simulink model "plant_n"  (R2023a)
settings: Solver=FixedStepAuto  StartTime=0.0  StopTime=200  FixedStep=0.01  RelTol=1e-3
values from neighbouring files (symbols this model uses):
  filter_3 = conv([0.1,1],conv([0.1 1],[0.1 1]))    [main_proj.m]
  filter_x = conv([0.7,1],conv([0.7 1],[0.7 1]))    [main_proj.m]
  kd = 1.117    [main_proj.m]
  ki = 4.47    [main_proj.m]
  kp = 5.366    [main_proj.m]
libraries: neural x772, slpidlib x6
(part 15 of 26)

== system plant_n/NARX Neural Network m8 gud (solution 2)/Layer 1/Delays 2 ==
  "p{1}" : Inport  PortDimensions=1  SampleTime=0.01
      mask Display: e = 0.06;c1 = [120 230 180]/255;c2 = ([120 230 180]+0)/(256+128);c3 = ([120 230 180]+128)/(256+128);patch([0 1 1 0],[0 0 1 1],c1);patch([0 1 1 1-e 1-e 0+e],[0 0 1 1-e 0+e 0+e],c2);patch([0 0 1 1-e 0+e 0+e],[0 1 1 1-e 1-e 0+e],c3);plot([0 1 1 0 0],[0 0 1 1 0]);
  Delay 1 : UnitDelay  InitialCondition=ai_layer_2_delayed_1  SampleTime=0.01
      mask Display: e = 0.06;c1 = [120 150 230]/255;c2 = ([120 150 230]+0)/383;c3 = ([120 150 230]+128)/383;patch([0 1 1 0],[0 0 1 1],c1);patch([0 1 1 1-e 1-e 0+e],[0 0 1 1-e 0+e 0+e],c2);patch([0 0 1 1-e 0+e 0+e],[0 1 1 1-e 1-e 0+e],c3);plot([0 1 1 0 0],[0 0 1 1 0]);disp('D')
  Delay 10 : UnitDelay  InitialCondition=ai_layer_2_delayed_10  SampleTime=0.01
      mask Display: e = 0.06;c1 = [120 150 230]/255;c2 = ([120 150 230]+0)/383;c3 = ([120 150 230]+128)/383;patch([0 1 1 0],[0 0 1 1],c1);patch([0 1 1 1-e 1-e 0+e],[0 0 1 1-e 0+e 0+e],c2);patch([0 0 1 1-e 0+e 0+e],[0 1 1 1-e 1-e 0+e],c3);plot([0 1 1 0 0],[0 0 1 1 0]);disp('D')
  Delay 11 : UnitDelay  InitialCondition=ai_layer_2_delayed_11  SampleTime=0.01
      mask Display: e = 0.06;c1 = [120 150 230]/255;c2 = ([120 150 230]+0)/383;c3 = ([120 150 230]+128)/383;patch([0 1 1 0],[0 0 1 1],c1);patch([0 1 1 1-e 1-e 0+e],[0 0 1 1-e 0+e 0+e],c2);patch([0 0 1 1-e 0+e 0+e],[0 1 1 1-e 1-e 0+e],c3);plot([0 1 1 0 0],[0 0 1 1 0]);disp('D')
  Delay 12 : UnitDelay  InitialCondition=ai_layer_2_delayed_12  SampleTime=0.01
      mask Display: e = 0.06;c1 = [120 150 230]/255;c2 = ([120 150 230]+0)/383;c3 = ([120 150 230]+128)/383;patch([0 1 1 0],[0 0 1 1],c1);patch([0 1 1 1-e 1-e 0+e],[0 0 1 1-e 0+e 0+e],c2);patch([0 0 1 1-e 0+e 0+e],[0 1 1 1-e 1-e 0+e],c3);plot([0 1 1 0 0],[0 0 1 1 0]);disp('D')
  Delay 2 : UnitDelay  InitialCondition=ai_layer_2_delayed_2  SampleTime=0.01
      mask Display: e = 0.06;c1 = [120 150 230]/255;c2 = ([120 150 230]+0)/383;c3 = ([120 150 230]+128)/383;patch([0 1 1 0],[0 0 1 1],c1);patch([0 1 1 1-e 1-e 0+e],[0 0 1 1-e 0+e 0+e],c2);patch([0 0 1 1-e 0+e 0+e],[0 1 1 1-e 1-e 0+e],c3);plot([0 1 1 0 0],[0 0 1 1 0]);disp('D')
  Delay 3 : UnitDelay  InitialCondition=ai_layer_2_delayed_3  SampleTime=0.01
      mask Display: e = 0.06;c1 = [120 150 230]/255;c2 = ([120 150 230]+0)/383;c3 = ([120 150 230]+128)/383;patch([0 1 1 0],[0 0 1 1],c1);patch([0 1 1 1-e 1-e 0+e],[0 0 1 1-e 0+e 0+e],c2);patch([0 0 1 1-e 0+e 0+e],[0 1 1 1-e 1-e 0+e],c3);plot([0 1 1 0 0],[0 0 1 1 0]);disp('D')
  Delay 4 : UnitDelay  InitialCondition=ai_layer_2_delayed_4  SampleTime=0.01
      mask Display: e = 0.06;c1 = [120 150 230]/255;c2 = ([120 150 230]+0)/383;c3 = ([120 150 230]+128)/383;patch([0 1 1 0],[0 0 1 1],c1);patch([0 1 1 1-e 1-e 0+e],[0 0 1 1-e 0+e 0+e],c2);patch([0 0 1 1-e 0+e 0+e],[0 1 1 1-e 1-e 0+e],c3);plot([0 1 1 0 0],[0 0 1 1 0]);disp('D')
  Delay 5 : UnitDelay  InitialCondition=ai_layer_2_delayed_5  SampleTime=0.01
      mask Display: e = 0.06;c1 = [120 150 230]/255;c2 = ([120 150 230]+0)/383;c3 = ([120 150 230]+128)/383;patch([0 1 1 0],[0 0 1 1],c1);patch([0 1 1 1-e 1-e 0+e],[0 0 1 1-e 0+e 0+e],c2);patch([0 0 1 1-e 0+e 0+e],[0 1 1 1-e 1-e 0+e],c3);plot([0 1 1 0 0],[0 0 1 1 0]);disp('D')
  Delay 6 : UnitDelay  InitialCondition=ai_layer_2_delayed_6  SampleTime=0.01
      mask Display: e = 0.06;c1 = [120 150 230]/255;c2 = ([120 150 230]+0)/383;c3 = ([120 150 230]+128)/383;patch([0 1 1 0],[0 0 1 1],c1);patch([0 1 1 1-e 1-e 0+e],[0 0 1 1-e 0+e 0+e],c2);patch([0 0 1 1-e 0+e 0+e],[0 1 1 1-e 1-e 0+e],c3);plot([0 1 1 0 0],[0 0 1 1 0]);disp('D')
  Delay 7 : UnitDelay  InitialCondition=ai_layer_2_delayed_7  SampleTime=0.01
      mask Display: e = 0.06;c1 = [120 150 230]/255;c2 = ([120 150 230]+0)/383;c3 = ([120 150 230]+128)/383;patch([0 1 1 0],[0 0 1 1],c1);patch([0 1 1 1-e 1-e 0+e],[0 0 1 1-e 0+e 0+e],c2);patch([0 0 1 1-e 0+e 0+e],[0 1 1 1-e 1-e 0+e],c3);plot([0 1 1 0 0],[0 0 1 1 0]);disp('D')
  Delay 8 : UnitDelay  InitialCondition=ai_layer_2_delayed_8  SampleTime=0.01
      mask Display: e = 0.06;c1 = [120 150 230]/255;c2 = ([120 150 230]+0)/383;c3 = ([120 150 230]+128)/383;patch([0 1 1 0],[0 0 1 1],c1);patch([0 1 1 1-e 1-e 0+e],[0 0 1 1-e 0+e 0+e],c2);patch([0 0 1 1-e 0+e 0+e],[0 1 1 1-e 1-e 0+e],c3);plot([0 1 1 0 0],[0 0 1 1 0]);disp('D')
  Delay 9 : UnitDelay  InitialCondition=ai_layer_2_delayed_9  SampleTime=0.01
      mask Display: e = 0.06;c1 = [120 150 230]/255;c2 = ([120 150 230]+0)/383;c3 = ([120 150 230]+128)/383;patch([0 1 1 0],[0 0 1 1],c1);patch([0 1 1 1-e 1-e 0+e],[0 0 1 1-e 0+e 0+e],c2);patch([0 0 1 1-e 0+e 0+e],[0 1 1 1-e 1-e 0+e],c3);plot([0 1 1 0 0],[0 0 1 1 0]);disp('D')
  mux : Mux  Inputs=12
      mask Display: e = 0.06;c1 = [120 150 230]/255;c2 = ([120 150 230]+0)/383;c3 = ([120 150 230]+128)/383;patch([0 1 1 0],[0 0 1 1],c1);patch([0 1 1 1-e 1-e 0+e],[0 0 1 1-e 0+e 0+e],c2);patch([0 0 1 1-e 0+e 0+e],[0 1 1 1-e 1-e 0+e],c3);plot([0 1 1 0 0],[0 0 1 1 0]);disp('Mux')
  "pd{1,2}" : Outport
      mask Display: e = 0.06;c1 = [120 230 180]/255;c2 = ([120 230 180]+0)/(256+128);c3 = ([120 230 180]+128)/(256+128);patch([0 1 1 0],[0 0 1 1],c1);patch([0 1 1 1-e 1-e 0+e],[0 0 1 1-e 0+e 0+e],c2);patch([0 0 1 1-e 0+e 0+e],[0 1 1 1-e 1-e 0+e],c3);plot([0 1 1 0 0],[0 0 1 1 0]);
  wires:
  "p{1}"/1 -> Delay 1/1
  Delay 1/1 -> Delay 2/1, mux/1
  Delay 2/1 -> Delay 3/1, mux/2
  Delay 3/1 -> Delay 4/1, mux/3
  Delay 4/1 -> Delay 5/1, mux/4
  Delay 5/1 -> Delay 6/1, mux/5
  Delay 6/1 -> Delay 7/1, mux/6
  Delay 7/1 -> Delay 8/1, mux/7
  Delay 8/1 -> Delay 9/1, mux/8
  Delay 9/1 -> Delay 10/1, mux/9
  Delay 10/1 -> Delay 11/1, mux/10
  Delay 11/1 -> Delay 12/1, mux/11
  Delay 12/1 -> mux/12
  mux/1 -> "pd{1,2}"/1

== system plant_n/NARX Neural Network m8 gud (solution 2)/Layer 1/IW{1,1} ==
  "pd{1,1}" : Inport  PortDimensions=12  SampleTime=0.01
      mask Display: e = 0.06;c1 = [120 230 180]/255;c2 = ([120 230 180]+0)/(256+128);c3 = ([120 230 180]+128)/(256+128);patch([0 1 1 0],[0 0 1 1],c1);patch([0 1 1 1-e 1-e 0+e],[0 0 1 1-e 0+e 0+e],c2);patch([0 0 1 1-e 0+e 0+e],[0 1 1 1-e 1-e 0+e],c3);plot([0 1 1 0 0],[0 0 1 1 0]);
  "IW{1,1}(1,:)'" : Constant  Value=[-0.56334830130879154364009764321963302791118621826171875;-0.357985255096524290774340215648408047854900360107421875;0.283427998989764062809371125695179216563701629638671875;-0.52727885493944259831522458625840954482555389404296875;-0.278331944433723055265517132284003309905529022216796875;-0.6037598769818128818798186330241151154041290283203125;-0.252123927832144156813143354156636632978916168212890625;0.28838201323591317049022109131328761577606201171875;-0.463874462662791253730887319761677645146846771240234375;0.27896573584558381764253454093704931437969207763671875;0.50570674204775212245976945268921554088592529296875;-0.007390079131495852320099526622243502060882747173309326171875]
      mask Display: e = 0.06;c1 = [120 150 230]/255;c2 = ([120 150 230]+0)/383;c3 = ([120 150 230]+128)/383;patch([0 1 1 0],[0 0 1 1],c1);patch([0 1 1 1-e 1-e 0+e],[0 0 1 1-e 0+e 0+e],c2);patch([0 0 1 1-e 0+e 0+e],[0 1 1 1-e 1-e 0+e],c3);plot([0 1 1 0 0],[0 0 1 1 0]);disp('Weights');
  "IW{1,1}(10,:)'" : Constant  Value=[-0.690275840744874802368258315254934132099151611328125;-0.79728617428333803385243072625598870217800140380859375;0.177674477339559488964226829921244643628597259521484375;0.09590570580940356582022587872415897436439990997314453125;-0.28801320297100974077153523467131890356540679931640625;-0.6833243170596807747330103666172362864017486572265625;-0.22435716680905526398959182188264094293117523193359375;-0.6840716937023392230088347787386737763881683349609375;-0.475131576981321190888962746612378396093845367431640625;-0.12182823067504509884084740178877837024629116058349609375;0.093487293354278244716937251723720692098140716552734375;0.74502502276723092666799175276537425816059112548828125]
      mask Display: e = 0.06;c1 = [120 150 230]/255;c2 = ([120 150 230]+0)/383;c3 = ([120 150 230]+128)/383;patch([0 1 1 0],[0 0 1 1],c1);patch([0 1 1 1-e 1-e 0+e],[0 0 1 1-e 0+e 0+e],c2);patch([0 0 1 1-e 0+e 0+e],[0 1 1 1-e 1-e 0+e],c3);plot([0 1 1 0 0],[0 0 1 1 0]);disp('Weights');
  "IW{1,1}(11,:)'" : Constant  Value=[0.020807334832183312089970428360174992121756076812744140625;-0.72362889068850300144930542955989949405193328857421875;-0.955254334663456550202909056679345667362213134765625;-0.204760678764603853974080038824467919766902923583984375;0.371667191189833878706139103087480179965496063232421875;-0.42938605762169246293780133783002384006977081298828125;-0.09146518961475048892229011698873364366590976715087890625;0.7516682707084567649502560016117058694362640380859375;0.722135567066211958575649987324140965938568115234375;0.2184070815776478491354595234952284954488277435302734375;0.69775866315792012262164689673227258026599884033203125;-0.8721778633994456964018127109738998115062713623046875]
      mask Display: e = 0.06;c1 = [120 150 230]/255;c2 = ([120 150 230]+0)/383;c3 = ([120 150 230]+128)/383;patch([0 1 1 0],[0 0 1 1],c1);patch([0 1 1 1-e 1-e 0+e],[0 0 1 1-e 0+e 0+e],c2);patch([0 0 1 1-e 0+e 0+e],[0 1 1 1-e 1-e 0+e],c3);plot([0 1 1 0 0],[0 0 1 1 0]);disp('Weights');
  "IW{1,1}(12,:)'" : Constant  Value=[-1.057018932574201652840883980388753116130828857421875;0.1693893839232068210254311679818783886730670928955078125;-0.85044934461662291536043767337105236947536468505859375;0.75838542598846381270760730330948717892169952392578125;0.50790235655985827012415256831445731222629547119140625;-0.0171384088579385092387941114111526985652744770050048828125;-0.428656473069752019799949493972235359251499176025390625;-0.16818090949152197932647823108709417283535003662109375;-0.8651226870069035346233476957422681152820587158203125;-0.5193860764043047861804325293633155524730682373046875;1.0594564649420614710351173926028423011302947998046875;-0.1817459257744392930877808112200000323355197906494140625]
      mask Display: e = 0.06;c1 = [120 150 230]/255;c2 = ([120 150 230]+0)/383;c3 = ([120 150 230]+128)/383;patch([0 1 1 0],[0 0 1 1],c1);patch([0 1 1 1-e 1-e 0+e],[0 0 1 1-e 0+e 0+e],c2);patch([0 0 1 1-e 0+e 0+e],[0 1 1 1-e 1-e 0+e],c3);plot([0 1 1 0 0],[0 0 1 1 0]);disp('Weights');
  "IW{1,1}(13,:)'" : Constant  Value=[-0.585951041167996233838266562088392674922943115234375;0.716915749185477846339153984445147216320037841796875;-0.23957537814192109149047382743447087705135345458984375;-0.8104595833058401144199933696654625236988067626953125;-0.30478478512946394207716593882651068270206451416015625;0.81104511509295296178834178135730326175689697265625;0.64501496872723074194055925545399077236652374267578125;-0.07076557953330718520046360708874999545514583587646484375;0.107786241446574726499108010102645494043827056884765625;0.262021628214974822146388078181189484894275665283203125;0.2077129224946279439922847132038441486656665802001953125;-0.33823196160467261517368342538247816264629364013671875]
      mask Display: e = 0.06;c1 = [120 150 230]/255;c2 = ([120 150 230]+0)/383;c3 = ([120 150 230]+128)/383;patch([0 1 1 0],[0 0 1 1],c1);patch([0 1 1 1-e 1-e 0+e],[0 0 1 1-e 0+e 0+e],c2);patch([0 0 1 1-e 0+e 0+e],[0 1 1 1-e 1-e 0+e],c3);plot([0 1 1 0 0],[0 0 1 1 0]);disp('Weights');
  "IW{1,1}(14,:)'" : Constant  Value=[-0.021926861772730621424898345139808952808380126953125;0.8906753535205587102296931334421969950199127197265625;-0.36976128212221792690428401328972540795803070068359375;-0.345367710616706846682433251771726645529270172119140625;-0.768790324260997248728699560160748660564422607421875;-0.219877322789279794346128937831963412463665008544921875;0.6049218279495220951247347329626791179180145263671875;-0.4412884606493763239853933555423282086849212646484375;0.05255967818845840022756732423658831976354122161865234375;-0.45907623086972570991548536767368204891681671142578125;0.6549992864126437108751588311861269176006317138671875;0.488129180308522148123984152334742248058319091796875]
      mask Display: e = 0.06;c1 = [120 150 230]/255;c2 = ([120 150 230]+0)/383;c3 = ([120 150 230]+128)/383;patch([0 1 1 0],[0 0 1 1],c1);patch([0 1 1 1-e 1-e 0+e],[0 0 1 1-e 0+e 0+e],c2);patch([0 0 1 1-e 0+e 0+e],[0 1 1 1-e 1-e 0+e],c3);plot([0 1 1 0 0],[0 0 1 1 0]);disp('Weights');
  "IW{1,1}(15,:)'" : Constant  Value=[0.46117641601221526226339619825012050569057464599609375;-0.0895345461376331475111811641909298487007617950439453125;0.328264117492681528620579456401173956692218780517578125;0.511917503541946761203007554286159574985504150390625;-0.801266579608470141948828313616104423999786376953125;0.451910735167512012111501462641172111034393310546875;-0.2188741480298032893170301349528017453849315643310546875;-0.6286657891340030612781220042961649596691131591796875;0.8327123535010105825904247467406094074249267578125;0.18255510716111655877824659910402260720729827880859375;-0.7387495430428596687733033832046203315258026123046875;-0.3072498793567366437429200232145376503467559814453125]
      mask Display: e = 0.06;c1 = [120 150 230]/255;c2 = ([120 150 230]+0)/383;c3 = ([120 150 230]+128)/383;patch([0 1 1 0],[0 0 1 1],c1);patch([0 1 1 1-e 1-e 0+e],[0 0 1 1-e 0+e 0+e],c2);patch([0 0 1 1-e 0+e 0+e],[0 1 1 1-e 1-e 0+e],c3);plot([0 1 1 0 0],[0 0 1 1 0]);disp('Weights');
  "IW{1,1}(2,:)'" : Constant  Value=[0.0787588482440988169042128674846026115119457244873046875;-0.71485237410952573444689051029854454100131988525390625;-0.261021462395077563645173768236418254673480987548828125;-0.77190171434430976393770151844364590942859649658203125;0.6192120004761527685133160048280842602252960205078125;0.276209900461571955521122845311765559017658233642578125;0.1564198465414966821018794007613905705511569976806640625;0.86245245324036023948366391778108663856983184814453125;-0.029228672295336245723351709102644235827028751373291015625;-0.29333393668341434246116250506020151078701019287109375;0.6675369234504946458486074334359727799892425537109375;-0.6078291827270627667445523911737836897373199462890625]
      mask Display: e = 0.06;c1 = [120 150 230]/255;c2 = ([120 150 230]+0)/383;c3 = ([120 150 230]+128)/383;patch([0 1 1 0],[0 0 1 1],c1);patch([0 1 1 1-e 1-e 0+e],[0 0 1 1-e 0+e 0+e],c2);patch([0 0 1 1-e 0+e 0+e],[0 1 1 1-e 1-e 0+e],c3);plot([0 1 1 0 0],[0 0 1 1 0]);disp('Weights');
  "IW{1,1}(3,:)'" : Constant  Value=[-0.76808344267437067554027407823014073073863983154296875;-0.55038788676150252054952716207480989396572113037109375;0.77459185718728151837098039322881959378719329833984375;-0.499350522556929854456342354751541279256343841552734375;-0.908047325048035869343721060431562364101409912109375;-0.287074786361956768576675358417560346424579620361328125;0.6404765001640833066431923725758679211139678955078125;0.78235408277472651139561321542714722454547882080078125;0.5997842926650067685301337405689992010593414306640625;-0.486908024680651141391507508160430006682872772216796875;0.62504559351542832157377915791585110127925872802734375;-0.1936118783901183137974300052519538439810276031494140625]
      mask Display: e = 0.06;c1 = [120 150 230]/255;c2 = ([120 150 230]+0)/383;c3 = ([120 150 230]+128)/383;patch([0 1 1 0],[0 0 1 1],c1);patch([0 1 1 1-e 1-e 0+e],[0 0 1 1-e 0+e 0+e],c2);patch([0 0 1 1-e 0+e 0+e],[0 1 1 1-e 1-e 0+e],c3);plot([0 1 1 0 0],[0 0 1 1 0]);disp('Weights');
  "IW{1,1}(4,:)'" : Constant  Value=[-0.82639420868754076554552057132241316139698028564453125;-0.276346036675341577559805728014907799661159515380859375;-0.54739563886299269501733988363412208855152130126953125;0.032969016201114260955495893767874804325401782989501953125;0.342569758428644621783831780703621916472911834716796875;-0.33994997710060104179063955598394386470317840576171875;0.91375881388352431233812467326060868799686431884765625;-0.331584671920007900691729219033732078969478607177734375;0.36714835048246918791647885882412083446979522705078125;-0.0846176892761831833666974489460699260234832763671875;-0.92592303920993701549235765924095176160335540771484375;-0.93601802735372918728984359404421411454677581787109375]
      mask Display: e = 0.06;c1 = [120 150 230]/255;c2 = ([120 150 230]+0)/383;c3 = ([120 150 230]+128)/383;patch([0 1 1 0],[0 0 1 1],c1);patch([0 1 1 1-e 1-e 0+e],[0 0 1 1-e 0+e 0+e],c2);patch([0 0 1 1-e 0+e 0+e],[0 1 1 1-e 1-e 0+e],c3);plot([0 1 1 0 0],[0 0 1 1 0]);disp('Weights');
  "IW{1,1}(5,:)'" : Constant  Value=[0.91859542281127726237599517844500951468944549560546875;-0.07037748658693605829927975037207943387329578399658203125;-0.8512540956376100087510394587297923862934112548828125;0.72619971995342369464054854688583873212337493896484375;0.720470041856829279680596300750039517879486083984375;-0.330330449866135189562754703729297034442424774169921875;-0.484010321857564485004132848189328797161579132080078125;-0.372095135170765367593759265218977816402912139892578125;0.521060814862327692509325061109848320484161376953125;0.63264959715850077603960244232439436018466949462890625;-0.432322011952695373082633523154072463512420654296875;0.499313726904651422611181033062166534364223480224609375]
      mask Display: e = 0.06;c1 = [120 150 230]/255;c2 = ([120 150 230]+0)/383;c3 = ([120 150 230]+128)/383;patch([0 1 1 0],[0 0 1 1],c1);patch([0 1 1 1-e 1-e 0+e],[0 0 1 1-e 0+e 0+e],c2);patch([0 0 1 1-e 0+e 0+e],[0 1 1 1-e 1-e 0+e],c3);plot([0 1 1 0 0],[0 0 1 1 0]);disp('Weights');
  "IW{1,1}(6,:)'" : Constant  Value=[0.93696082681236714240213814264279790222644805908203125;-0.27588909036586650724842684212489984929561614990234375;-0.6889927007440055373166387653327547013759613037109375;0.85547503643398348227577798752463422715663909912109375;-0.7718420202962541498692417007987387478351593017578125;-0.9429513036639611822664619467104785144329071044921875;-0.8577089563521986814720321490312926471233367919921875;0.8899270804914698462795286104665137827396392822265625;0.443109597734193616513920233046519570052623748779296875;1.0531520200119077745881668306537903845310211181640625;-0.2175598841645387249155163544855895452201366424560546875;-0.72738179658011070660705854606931097805500030517578125]
      mask Display: e = 0.06;c1 = [120 150 230]/255;c2 = ([120 150 230]+0)/383;c3 = ([120 150 230]+128)/383;patch([0 1 1 0],[0 0 1 1],c1);patch([0 1 1 1-e 1-e 0+e],[0 0 1 1-e 0+e 0+e],c2);patch([0 0 1 1-e 0+e 0+e],[0 1 1 1-e 1-e 0+e],c3);plot([0 1 1 0 0],[0 0 1 1 0]);disp('Weights');
  "IW{1,1}(7,:)'" : Constant  Value=[0.317539016680124686065056494044256396591663360595703125;-0.6484067800480979304467155088786967098712921142578125;-0.330605962287668309063093374788877554237842559814453125;0.56710250888755597831192289959290064871311187744140625;0.298819571483376400511389192615752108395099639892578125;0.60228092181639902857881452291621826589107513427734375;-0.6607813044442212291329497020342387259006500244140625;-0.4153000444487464637433049574610777199268341064453125;-0.621645882898536950023071767645888030529022216796875;0.07232726468850238232821681094719679094851016998291015625;-0.0235717249783840600285689248494236380793154239654541015625;0.692179622775543901269656998920254409313201904296875]
      mask Display: e = 0.06;c1 = [120 150 230]/255;c2 = ([120 150 230]+0)/383;c3 = ([120 150 230]+128)/383;patch([0 1 1 0],[0 0 1 1],c1);patch([0 1 1 1-e 1-e 0+e],[0 0 1 1-e 0+e 0+e],c2);patch([0 0 1 1-e 0+e 0+e],[0 1 1 1-e 1-e 0+e],c3);plot([0 1 1 0 0],[0 0 1 1 0]);disp('Weights');
  "IW{1,1}(8,:)'" : Constant  Value=[0.08781056476112426845137548525599413551390171051025390625;-0.91916651525158987734442916917032562196254730224609375;0.36400432919801506415069525246508419513702392578125;-0.75661023144707806320496956686838530004024505615234375;-0.83966916109414324598247958419960923492908477783203125;0.28422364194135651960237964885891415178775787353515625;-0.0149951949502383496959367903400561772286891937255859375;-0.362236545882393123907405652062152512371540069580078125;-0.94172749823212209552281137803220190107822418212890625;-0.47474571884634120255697098400560207664966583251953125;0.42822215133623675598073532455600798130035400390625;0.91691101236875294233641398022882640361785888671875]
      mask Display: e = 0.06;c1 = [120 150 230]/255;c2 = ([120 150 230]+0)/383;c3 = ([120 150 230]+128)/383;patch([0 1 1 0],[0 0 1 1],c1);patch([0 1 1 1-e 1-e 0+e],[0 0 1 1-e 0+e 0+e],c2);patch([0 0 1 1-e 0+e 0+e],[0 1 1 1-e 1-e 0+e],c3);plot([0 1 1 0 0],[0 0 1 1 0]);disp('Weights');
  "IW{1,1}(9,:)'" : Constant  Value=[0.516648633279290780961900964030064642429351806640625;0.79527388990046798955546591969323344528675079345703125;-0.73508776086802363192163056737626902759075164794921875;0.66175699013347377697158435694291256368160247802734375;-0.9491096813545978339021758074522949755191802978515625;-0.410442549438077064483110234505147673189640045166015625;-0.423362511508447780794739401244441978633403778076171875;-0.7672771910530207239986566492007113993167877197265625;-0.0754615582126294537346211654949001967906951904296875;-0.343839991961225444061511780091677792370319366455078125;0.15150606718300518860331749237957410514354705810546875;0.0806243665767537864841330019771703518927097320556640625]
      mask Display: e = 0.06;c1 = [120 150 230]/255;c2 = ([120 150 230]+0)/383;c3 = ([120 150 230]+128)/383;patch([0 1 1 0],[0 0 1 1],c1);patch([0 1 1 1-e 1-e 0+e],[0 0 1 1-e 0+e 0+e],c2);patch([0 0 1 1-e 0+e 0+e],[0 1 1 1-e 1-e 0+e],c3);plot([0 1 1 0 0],[0 0 1 1 0]);disp('Weights');
  Mux : Mux  Inputs=15
      mask Display: e = 0.06;c1 = [120 150 230]/255;c2 = ([120 150 230]+0)/383;c3 = ([120 150 230]+128)/383;patch([0 1 1 0],[0 0 1 1],c1);patch([0 1 1 1-e 1-e 0+e],[0 0 1 1-e 0+e 0+e],c2);patch([0 0 1 1-e 0+e 0+e],[0 1 1 1-e 1-e 0+e],c3);plot([0 1 1 0 0],[0 0 1 1 0]);disp('Mux');
  dotprod{1..15} (15 alike) : neural/Weight Functions/dotprod
  "iz{1,1}" : Outport
      mask Display: e = 0.06;c1 = [120 230 180]/255;c2 = ([120 230 180]+0)/(256+128);c3 = ([120 230 180]+128)/(256+128);patch([0 1 1 0],[0 0 1 1],c1);patch([0 1 1 1-e 1-e 0+e],[0 0 1 1-e 0+e 0+e],c2);patch([0 0 1 1-e 0+e 0+e],[0 1 1 1-e 1-e 0+e],c3);plot([0 1 1 0 0],[0 0 1 1 0]);
  wires:
  "IW{1,1}(1,:)'"/1 -> dotprod1/1
  "pd{1,1}"/1 -> dotprod1/2, dotprod2/2, dotprod3/2, dotprod4/2, dotprod5/2, dotprod6/2, dotprod7/2, dotprod8/2, dotprod9/2, dotprod10/2, dotprod11/2, dotprod12/2, dotprod13/2, dotprod14/2, dotprod15/2
  dotprod1/1 -> Mux/1
  "IW{1,1}(2,:)'"/1 -> dotprod2/1
  dotprod2/1 -> Mux/2
  "IW{1,1}(3,:)'"/1 -> dotprod3/1
  dotprod3/1 -> Mux/3
  "IW{1,1}(4,:)'"/1 -> dotprod4/1
  dotprod4/1 -> Mux/4
  "IW{1,1}(5,:)'"/1 -> dotprod5/1
  dotprod5/1 -> Mux/5
  "IW{1,1}(6,:)'"/1 -> dotprod6/1
  dotprod6/1 -> Mux/6
  "IW{1,1}(7,:)'"/1 -> dotprod7/1
  dotprod7/1 -> Mux/7
  "IW{1,1}(8,:)'"/1 -> dotprod8/1
  dotprod8/1 -> Mux/8
  "IW{1,1}(9,:)'"/1 -> dotprod9/1
  dotprod9/1 -> Mux/9
  "IW{1,1}(10,:)'"/1 -> dotprod10/1
  dotprod10/1 -> Mux/10
  "IW{1,1}(11,:)'"/1 -> dotprod11/1
  dotprod11/1 -> Mux/11
  "IW{1,1}(12,:)'"/1 -> dotprod12/1
  dotprod12/1 -> Mux/12
  "IW{1,1}(13,:)'"/1 -> dotprod13/1
  dotprod13/1 -> Mux/13
  "IW{1,1}(14,:)'"/1 -> dotprod14/1
  dotprod14/1 -> Mux/14
  "IW{1,1}(15,:)'"/1 -> dotprod15/1
  dotprod15/1 -> Mux/15
  Mux/1 -> "iz{1,1}"/1

== system plant_n/NARX Neural Network m8 gud (solution 2)/Layer 1/LW{1,2} ==
  "ad{1,2}" : Inport  PortDimensions=12  SampleTime=0.01
      mask Display: e = 0.06;c1 = [120 230 180]/255;c2 = ([120 230 180]+0)/(256+128);c3 = ([120 230 180]+128)/(256+128);patch([0 1 1 0],[0 0 1 1],c1);patch([0 1 1 1-e 1-e 0+e],[0 0 1 1-e 0+e 0+e],c2);patch([0 0 1 1-e 0+e 0+e],[0 1 1 1-e 1-e 0+e],c3);plot([0 1 1 0 0],[0 0 1 1 0]);
  "IW{1,2}(1,:)'" : Constant  Value=[-1.106579679929702297869198446278460323810577392578125;0.52825754089354981513082520905300043523311614990234375;-0.209788113019308275486451975666568614542484283447265625;-0.70460030462073708346082412390387617051601409912109375;-0.401771680824487831262814552246709354221820831298828125;0.65111397584809693750429460123996250331401824951171875;0.99474516526987499798195813127676956355571746826171875;0.14611346021854132448680729794432409107685089111328125;-0.269030442825935744988186115733697079122066497802734375;-0.468383848704074068347580350746284238994121551513671875;-0.022538785323445019448396209327256656251847743988037109375;-0.1965076576250255058209148728565196506679058074951171875]
      mask Display: e = 0.06;c1 = [120 150 230]/255;c2 = ([120 150 230]+0)/383;c3 = ([120 150 230]+128)/383;patch([0 1 1 0],[0 0 1 1],c1);patch([0 1 1 1-e 1-e 0+e],[0 0 1 1-e 0+e 0+e],c2);patch([0 0 1 1-e 0+e 0+e],[0 1 1 1-e 1-e 0+e],c3);plot([0 1 1 0 0],[0 0 1 1 0]);disp('weights');
  "IW{1,2}(10,:)'" : Constant  Value=[-0.1766532618747101712752822777474648319184780120849609375;-0.3745556692362317363631518674083054065704345703125;-0.1144474116627141047075610913452692329883575439453125;0.20949512269696379807015773621969856321811676025390625;-0.03906938417347492753517457231282605789601802825927734375;0.2115180890305794758621260598374647088348865509033203125;-0.2816719455949272532535587743041105568408966064453125;0.62025766970232376618099578990950249135494232177734375;0.391590978897741859299230782198719680309295654296875;-0.326766475024203806309941455765510909259319305419921875;0.483595620121272329328121486469171941280364990234375;-0.50076224588811435456392473497544415295124053955078125]
      mask Display: e = 0.06;c1 = [120 150 230]/255;c2 = ([120 150 230]+0)/383;c3 = ([120 150 230]+128)/383;patch([0 1 1 0],[0 0 1 1],c1);patch([0 1 1 1-e 1-e 0+e],[0 0 1 1-e 0+e 0+e],c2);patch([0 0 1 1-e 0+e 0+e],[0 1 1 1-e 1-e 0+e],c3);plot([0 1 1 0 0],[0 0 1 1 0]);disp('weights');
  "IW{1,2}(11,:)'" : Constant  Value=[1.2592430139325150317830548374331556260585784912109375;-0.05691356119298808524664678998306044377386569976806640625;0.77803559816210843269601582505856640636920928955078125;-0.491208868074326954200614636647514998912811279296875;-0.51505931328393550483468743550474755465984344482421875;0.420311168434700010987370433213072828948497772216796875;0.024502453613158510503655662660094094462692737579345703125;0.1425078536734706580180187529549584724009037017822265625;-0.80727339564517619496797351530403830111026763916015625;-0.5388962635981133786344798863865435123443603515625;-0.213317811245898714123114814356085844337940216064453125;0.51164862064301541710875653734547086060047149658203125]
      mask Display: e = 0.06;c1 = [120 150 230]/255;c2 = ([120 150 230]+0)/383;c3 = ([120 150 230]+128)/383;patch([0 1 1 0],[0 0 1 1],c1);patch([0 1 1 1-e 1-e 0+e],[0 0 1 1-e 0+e 0+e],c2);patch([0 0 1 1-e 0+e 0+e],[0 1 1 1-e 1-e 0+e],c3);plot([0 1 1 0 0],[0 0 1 1 0]);disp('weights');
  "IW{1,2}(12,:)'" : Constant  Value=[0.2144743579478212980315987579160719178617000579833984375;0.367636065286543967101096086480538360774517059326171875;-0.424155526317948339265484491988900117576122283935546875;-0.6061814219902481593038601204170845448970794677734375;-0.09018792250183350900361034518937231041491031646728515625;-0.0293812933567908218801534303565858863294124603271484375;0.70801196688227985287511501155677251517772674560546875;0.91311583202700641326288177879177965223789215087890625;0.58870276977829794073926450437284074723720550537109375;0.52471984726705345192243612473248504102230072021484375;-0.41813703421421222206078027738840319216251373291015625;-0.627176786045356760013191887992434203624725341796875]
      mask Display: e = 0.06;c1 = [120 150 230]/255;c2 = ([120 150 230]+0)/383;c3 = ([120 150 230]+128)/383;patch([0 1 1 0],[0 0 1 1],c1);patch([0 1 1 1-e 1-e 0+e],[0 0 1 1-e 0+e 0+e],c2);patch([0 0 1 1-e 0+e 0+e],[0 1 1 1-e 1-e 0+e],c3);plot([0 1 1 0 0],[0 0 1 1 0]);disp('weights');
  "IW{1,2}(13,:)'" : Constant  Value=[-0.83153955411432145528038972770445980131626129150390625;0.259968350632096445451679755933582782745361328125;0.5642431152716707032368503860197961330413818359375;0.5656525432028589595034873127588070929050445556640625;0.79903642750351966395072622617590241134166717529296875;0.854598651285486621276277219294570386409759521484375;0.2405362118651295511018162187610869295895099639892578125;-0.308453932417994014514306400087662041187286376953125;-0.81404087650358913919035330764017999172210693359375;-0.58749999584968026766773618874140083789825439453125;-0.290260874324910045363168364929151721298694610595703125;-0.419206670436782447008994267889647744596004486083984375]
      mask Display: e = 0.06;c1 = [120 150 230]/255;c2 = ([120 150 230]+0)/383;c3 = ([120 150 230]+128)/383;patch([0 1 1 0],[0 0 1 1],c1);patch([0 1 1 1-e 1-e 0+e],[0 0 1 1-e 0+e 0+e],c2);patch([0 0 1 1-e 0+e 0+e],[0 1 1 1-e 1-e 0+e],c3);plot([0 1 1 0 0],[0 0 1 1 0]);disp('weights');
  "IW{1,2}(14,:)'" : Constant  Value=[0.932479306092938831085348283522762358188629150390625;-0.0272475041537409527758750726889047655276954174041748046875;0.58201983329524742405425286051467992365360260009765625;0.56306687430555324436198816329124383628368377685546875;-0.115604398118128892658518225289299152791500091552734375;0.221592492699736631767137851056759245693683624267578125;0.30149571316118206620870978440507315099239349365234375;-0.52733065035402770792671844901633448898792266845703125;-0.32289354256519520181001325909164734184741973876953125;0.26418510460360311586924808580079115927219390869140625;0.451534475019637449033638176842941902577877044677734375;0.490157427082875518653537483260151930153369903564453125]
      mask Display: e = 0.06;c1 = [120 150 230]/255;c2 = ([120 150 230]+0)/383;c3 = ([120 150 230]+128)/383;patch([0 1 1 0],[0 0 1 1],c1);patch([0 1 1 1-e 1-e 0+e],[0 0 1 1-e 0+e 0+e],c2);patch([0 0 1 1-e 0+e 0+e],[0 1 1 1-e 1-e 0+e],c3);plot([0 1 1 0 0],[0 0 1 1 0]);disp('weights');
  "IW{1,2}(15,:)'" : Constant  Value=[0.54023941275809317374978490988723933696746826171875;0.70538843084802149707712715098750777542591094970703125;0.126661458442705543436801463030860759317874908447265625;0.1296631038325960771917522151852608658373355865478515625;-0.831707942749137174587303888984024524688720703125;0.3484679551356018034624639767571352422237396240234375;-0.65556879555840119611076488581602461636066436767578125;0.71725999512402827118506820625043474137783050537109375;0.6103413533630241971650320920161902904510498046875;-0.883064273610031147399013207177631556987762451171875;1.1450447317144922809717400014051236212253570556640625;0.398361915904074936900514103399473242461681365966796875]
      mask Display: e = 0.06;c1 = [120 150 230]/255;c2 = ([120 150 230]+0)/383;c3 = ([120 150 230]+128)/383;patch([0 1 1 0],[0 0 1 1],c1);patch([0 1 1 1-e 1-e 0+e],[0 0 1 1-e 0+e 0+e],c2);patch([0 0 1 1-e 0+e 0+e],[0 1 1 1-e 1-e 0+e],c3);plot([0 1 1 0 0],[0 0 1 1 0]);disp('weights');
  "IW{1,2}(2,:)'" : Constant  Value=[-0.0613607485209021474847901345128775574266910552978515625;0.2102986317005552663328415974319796077907085418701171875;0.51227340316594638380820470047183334827423095703125;-0.4384509371626512663766561672673560678958892822265625;-0.58884444650935729992369260799023322761058807373046875;-0.6952179252414676380311675529810599982738494873046875;-0.0453869724025333376449253819373552687466144561767578125;-0.54671910234365128644640208221971988677978515625;-0.1725543729219697619559070744799100793898105621337890625;-0.06524493320775152926938034170234459452331066131591796875;1.0870171743383616469458274877979420125484466552734375;1.1102624429816270179571802145801484584808349609375]
      mask Display: e = 0.06;c1 = [120 150 230]/255;c2 = ([120 150 230]+0)/383;c3 = ([120 150 230]+128)/383;patch([0 1 1 0],[0 0 1 1],c1);patch([0 1 1 1-e 1-e 0+e],[0 0 1 1-e 0+e 0+e],c2);patch([0 0 1 1-e 0+e 0+e],[0 1 1 1-e 1-e 0+e],c3);plot([0 1 1 0 0],[0 0 1 1 0]);disp('weights');
  "IW{1,2}(3,:)'" : Constant  Value=[-0.80344702836685721880627397695207037031650543212890625;0.6060054586593153214124640726367942988872528076171875;0.94174433355452691341014315185020677745342254638671875;-0.45769314793643622873986487320507876574993133544921875;1.0271665041981450361419092587311752140522003173828125;-0.323454616684653528668746957919211126863956451416015625;-0.79136388342700125786421949669602327048778533935546875;-0.70599310373184842593019538981025107204914093017578125;0.52276401571592912009833753472776152193546295166015625;-0.336390838337624009657389478888944722712039947509765625;-0.80549047063324252793137247863342054188251495361328125;-0.53559323045169471289028706451063044369220733642578125]
      mask Display: e = 0.06;c1 = [120 150 230]/255;c2 = ([120 150 230]+0)/383;c3 = ([120 150 230]+128)/383;patch([0 1 1 0],[0 0 1 1],c1);patch([0 1 1 1-e 1-e 0+e],[0 0 1 1-e 0+e 0+e],c2);patch([0 0 1 1-e 0+e 0+e],[0 1 1 1-e 1-e 0+e],c3);plot([0 1 1 0 0],[0 0 1 1 0]);disp('weights');
  "IW{1,2}(4,:)'" : Constant  Value=[-0.7426673256625624386373374363756738603115081787109375;-0.74682544445321685788741206124541349709033966064453125;-0.734244610304327860461626187316142022609710693359375;-0.30407297409185929382147151045501232147216796875;0.1945728148567196225116049390635453164577484130859375;0.08330616560221947020092869706786586903035640716552734375;-0.70236392908091305198325926539837382733821868896484375;0.8314744072967445998045832311618141829967498779296875;0.467643630495797157919923847657628357410430908203125;-0.5198915802764181304240764802671037614345550537109375;-0.323876652776586393400748420390300452709197998046875;-0.4744635837454687088410310025210492312908172607421875]
      mask Display: e = 0.06;c1 = [120 150 230]/255;c2 = ([120 150 230]+0)/383;c3 = ([120 150 230]+128)/383;patch([0 1 1 0],[0 0 1 1],c1);patch([0 1 1 1-e 1-e 0+e],[0 0 1 1-e 0+e 0+e],c2);patch([0 0 1 1-e 0+e 0+e],[0 1 1 1-e 1-e 0+e],c3);plot([0 1 1 0 0],[0 0 1 1 0]);disp('weights');
  "IW{1,2}(5,:)'" : Constant  Value=[-0.812688840936343748211356796673499047756195068359375;-0.2327481448855746315462766915516112931072711944580078125;-0.077693909908231939542844202151172794401645660400390625;0.61947138286000880125214962390600703656673431396484375;-0.61216356229057711235697070151218213140964508056640625;0.1402599969088374198822322114210692234337329864501953125;-0.251025670461214212014766644642804749310016632080078125;0.471971295926272238485665866392082534730434417724609375;-0.11707983728669839329494806179354782216250896453857421875;0.35985519858911996227135432491195388138294219970703125;-0.144352563596631233711065078750834800302982330322265625;0.1597679980000514532445521354020456783473491668701171875]
      mask Display: e = 0.06;c1 = [120 150 230]/255;c2 = ([120 150 230]+0)/383;c3 = ([120 150 230]+128)/383;patch([0 1 1 0],[0 0 1 1],c1);patch([0 1 1 1-e 1-e 0+e],[0 0 1 1-e 0+e 0+e],c2);patch([0 0 1 1-e 0+e 0+e],[0 1 1 1-e 1-e 0+e],c3);plot([0 1 1 0 0],[0 0 1 1 0]);disp('weights');
  "IW{1,2}(6,:)'" : Constant  Value=[0.98991897750220469998083672180655412375926971435546875;-0.482706050830979283006172408931888639926910400390625;-0.85313013555683692157316500015440396964550018310546875;0.40972106976131872357882457436062395572662353515625;0.379758904813073616679730548639781773090362548828125;-0.53356366489194584357136363905738107860088348388671875;-0.11211290106695158408367518632076098583638668060302734375;0.15559924442930206378576940551283769309520721435546875;0.74662046515104474320168037593248300254344940185546875;-0.371698578092490683477677748669520951807498931884765625;-0.539680004349044839528914963011629879474639892578125;-0.403504549029664427717278840646031312644481658935546875]
      mask Display: e = 0.06;c1 = [120 150 230]/255;c2 = ([120 150 230]+0)/383;c3 = ([120 150 230]+128)/383;patch([0 1 1 0],[0 0 1 1],c1);patch([0 1 1 1-e 1-e 0+e],[0 0 1 1-e 0+e 0+e],c2);patch([0 0 1 1-e 0+e 0+e],[0 1 1 1-e 1-e 0+e],c3);plot([0 1 1 0 0],[0 0 1 1 0]);disp('weights');
  "IW{1,2}(7,:)'" : Constant  Value=[0.22118631392469456642402292345650494098663330078125;0.759031077557348776707613069447688758373260498046875;0.0915195665891657961221739014945342205464839935302734375;0.8388678429358342736321674237842671573162078857421875;-0.321082401091234037604493778417236171662807464599609375;-0.366299073638256533769208544981665909290313720703125;-0.7830827258622143904887025200878269970417022705078125;0.82954652938512485338407032031682319939136505126953125;0.2443994290634696475716935992750222794711589813232421875;-0.6714107782201332863536435979767702519893646240234375;0.1129331912517489711067497637486667372286319732666015625;0.2786128071999389721469242431339807808399200439453125]
      mask Display: e = 0.06;c1 = [120 150 230]/255;c2 = ([120 150 230]+0)/383;c3 = ([120 150 230]+128)/383;patch([0 1 1 0],[0 0 1 1],c1);patch([0 1 1 1-e 1-e 0+e],[0 0 1 1-e 0+e 0+e],c2);patch([0 0 1 1-e 0+e 0+e],[0 1 1 1-e 1-e 0+e],c3);plot([0 1 1 0 0],[0 0 1 1 0]);disp('weights');
  "IW{1,2}(8,:)'" : Constant  Value=[-0.07696744006295107298765145742436288855969905853271484375;0.9417715107075468328190481770434416830539703369140625;-0.31577273176542608457140204336610622704029083251953125;0.7905628230298968883715815536561422049999237060546875;0.77146155564474450105905134478234685957431793212890625;-0.5572470094687627106821992128971032798290252685546875;0.1505089879695258592295914468195405788719654083251953125;0.422473482469485961399158213680493645370006561279296875;0.32430131586564658885407652633148245513439178466796875;-0.389208775052764632818025347660295665264129638671875;0.935567966004068107821467492613010108470916748046875;-0.250288277024981631324607178612495772540569305419921875]
      mask Display: e = 0.06;c1 = [120 150 230]/255;c2 = ([120 150 230]+0)/383;c3 = ([120 150 230]+128)/383;patch([0 1 1 0],[0 0 1 1],c1);patch([0 1 1 1-e 1-e 0+e],[0 0 1 1-e 0+e 0+e],c2);patch([0 0 1 1-e 0+e 0+e],[0 1 1 1-e 1-e 0+e],c3);plot([0 1 1 0 0],[0 0 1 1 0]);disp('weights');
  "IW{1,2}(9,:)'" : Constant  Value=[0.75534181939414291040435500690364278852939605712890625;-0.2454563692478407277430818567154346965253353118896484375;-0.386275461184592494578993182585691101849079132080078125;0.07452799775149744621050018622554489411413669586181640625;-0.15830103094245140393780957310809753835201263427734375;0.62265927393231745856638781333458609879016876220703125;0.5855871920073172365306390929617919027805328369140625;-0.81654961874373321872866426929249428212642669677734375;-0.60594759429125655270098604887607507407665252685546875;0.73798974914088943943824006055365316569805145263671875;-0.479352570645532105597652616779669187963008880615234375;0.7670514996942709995408904433134011924266815185546875]
      mask Display: e = 0.06;c1 = [120 150 230]/255;c2 = ([120 150 230]+0)/383;c3 = ([120 150 230]+128)/383;patch([0 1 1 0],[0 0 1 1],c1);patch([0 1 1 1-e 1-e 0+e],[0 0 1 1-e 0+e 0+e],c2);patch([0 0 1 1-e 0+e 0+e],[0 1 1 1-e 1-e 0+e],c3);plot([0 1 1 0 0],[0 0 1 1 0]);disp('weights');
  Mux : Mux  Inputs=15
      mask Display: e = 0.06;c1 = [120 150 230]/255;c2 = ([120 150 230]+0)/383;c3 = ([120 150 230]+128)/383;patch([0 1 1 0],[0 0 1 1],c1);patch([0 1 1 1-e 1-e 0+e],[0 0 1 1-e 0+e 0+e],c2);patch([0 0 1 1-e 0+e 0+e],[0 1 1 1-e 1-e 0+e],c3);plot([0 1 1 0 0],[0 0 1 1 0]);disp('Mux');
  dotprod{1..15} (15 alike) : neural/Weight Functions/dotprod
  "lz{1,2}" : Outport
      mask Display: e = 0.06;c1 = [120 230 180]/255;c2 = ([120 230 180]+0)/(256+128);c3 = ([120 230 180]+128)/(256+128);patch([0 1 1 0],[0 0 1 1],c1);patch([0 1 1 1-e 1-e 0+e],[0 0 1 1-e 0+e 0+e],c2);patch([0 0 1 1-e 0+e 0+e],[0 1 1 1-e 1-e 0+e],c3);plot([0 1 1 0 0],[0 0 1 1 0]);
  wires:
  "IW{1,2}(1,:)'"/1 -> dotprod1/1
  "ad{1,2}"/1 -> dotprod1/2, dotprod2/2, dotprod3/2, dotprod4/2, dotprod5/2, dotprod6/2, dotprod7/2, dotprod8/2, dotprod9/2, dotprod10/2, dotprod11/2, dotprod12/2, dotprod13/2, dotprod14/2, dotprod15/2
  dotprod1/1 -> Mux/1
  "IW{1,2}(2,:)'"/1 -> dotprod2/1
  dotprod2/1 -> Mux/2
  "IW{1,2}(3,:)'"/1 -> dotprod3/1
  dotprod3/1 -> Mux/3
  "IW{1,2}(4,:)'"/1 -> dotprod4/1
  dotprod4/1 -> Mux/4
  "IW{1,2}(5,:)'"/1 -> dotprod5/1
  dotprod5/1 -> Mux/5
  "IW{1,2}(6,:)'"/1 -> dotprod6/1
  dotprod6/1 -> Mux/6
  "IW{1,2}(7,:)'"/1 -> dotprod7/1
  dotprod7/1 -> Mux/7
  "IW{1,2}(8,:)'"/1 -> dotprod8/1
  dotprod8/1 -> Mux/8
  "IW{1,2}(9,:)'"/1 -> dotprod9/1
  dotprod9/1 -> Mux/9
  "IW{1,2}(10,:)'"/1 -> dotprod10/1
  dotprod10/1 -> Mux/10
  "IW{1,2}(11,:)'"/1 -> dotprod11/1
  dotprod11/1 -> Mux/11
  "IW{1,2}(12,:)'"/1 -> dotprod12/1
  dotprod12/1 -> Mux/12
  "IW{1,2}(13,:)'"/1 -> dotprod13/1
  dotprod13/1 -> Mux/13
  "IW{1,2}(14,:)'"/1 -> dotprod14/1
  dotprod14/1 -> Mux/14
  "IW{1,2}(15,:)'"/1 -> dotprod15/1
  dotprod15/1 -> Mux/15
  Mux/1 -> "lz{1,2}"/1

== system plant_n/NARX Neural Network m8 gud (solution 2)/Layer 2/Delays 1 ==
  "p{2}" : Inport  PortDimensions=15  SampleTime=0.01
      mask Display: e = 0.06;c1 = [120 230 180]/255;c2 = ([120 230 180]+0)/(256+128);c3 = ([120 230 180]+128)/(256+128);patch([0 1 1 0],[0 0 1 1],c1);patch([0 1 1 1-e 1-e 0+e],[0 0 1 1-e 0+e 0+e],c2);patch([0 0 1 1-e 0+e 0+e],[0 1 1 1-e 1-e 0+e],c3);plot([0 1 1 0 0],[0 0 1 1 0]);
  mux : Mux  Inputs=1
      mask Display: e = 0.06;c1 = [120 150 230]/255;c2 = ([120 150 230]+0)/383;c3 = ([120 150 230]+128)/383;patch([0 1 1 0],[0 0 1 1],c1);patch([0 1 1 1-e 1-e 0+e],[0 0 1 1-e 0+e 0+e],c2);patch([0 0 1 1-e 0+e 0+e],[0 1 1 1-e 1-e 0+e],c3);plot([0 1 1 0 0],[0 0 1 1 0]);disp('Mux')
  "pd{2,1}" : Outport
      mask Display: e = 0.06;c1 = [120 230 180]/255;c2 = ([120 230 180]+0)/(256+128);c3 = ([120 230 180]+128)/(256+128);patch([0 1 1 0],[0 0 1 1],c1);patch([0 1 1 1-e 1-e 0+e],[0 0 1 1-e 0+e 0+e],c2);patch([0 0 1 1-e 0+e 0+e],[0 1 1 1-e 1-e 0+e],c3);plot([0 1 1 0 0],[0 0 1 1 0]);
  wires:
  "p{2}"/1 -> mux/1
  mux/1 -> "pd{2,1}"/1

== system plant_n/NARX Neural Network m8 gud (solution 2)/Layer 2/LW{2,1} ==
  "ad{2,1}" : Inport  PortDimensions=15  SampleTime=0.01
      mask Display: e = 0.06;c1 = [120 230 180]/255;c2 = ([120 230 180]+0)/(256+128);c3 = ([120 230 180]+128)/(256+128);patch([0 1 1 0],[0 0 1 1],c1);patch([0 1 1 1-e 1-e 0+e],[0 0 1 1-e 0+e 0+e],c2);patch([0 0 1 1-e 0+e 0+e],[0 1 1 1-e 1-e 0+e],c3);plot([0 1 1 0 0],[0 0 1 1 0]);
  "IW{2,1}(1,:)'" : Constant  Value=[-0.0683696139528004731555910211682203225791454315185546875;-0.342077040767760631734262233294430188834667205810546875;-0.1898921001033294364557235667234635911881923675537109375;-0.0134991569092649844885389853743618004955351352691650390625;-0.276242655581969198674840981766465120017528533935546875;-0.0394900299133619514524440319291898049414157867431640625;0.051075290526696050241728386254180804826319217681884765625;0.0900553514598873283691915503368363715708255767822265625;-0.129383778470535393267937251948751509189605712890625;-0.11903657915148881107914036192596540786325931549072265625;0.34242681736146585169677791782305575907230377197265625;-0.059843751373246899250002428516381769441068172454833984375;-0.1748916236651742173169310490266070701181888580322265625;0.1044461039262105928049351177833159454166889190673828125;-0.0309445952612202902776150637009777710773050785064697265625]
      mask Display: e = 0.06;c1 = [120 150 230]/255;c2 = ([120 150 230]+0)/383;c3 = ([120 150 230]+128)/383;patch([0 1 1 0],[0 0 1 1],c1);patch([0 1 1 1-e 1-e 0+e],[0 0 1 1-e 0+e 0+e],c2);patch([0 0 1 1-e 0+e 0+e],[0 1 1 1-e 1-e 0+e],c3);plot([0 1 1 0 0],[0 0 1 1 0]);disp('weights');
  Mux : Mux  Inputs=1
      mask Display: e = 0.06;c1 = [120 150 230]/255;c2 = ([120 150 230]+0)/383;c3 = ([120 150 230]+128)/383;patch([0 1 1 0],[0 0 1 1],c1);patch([0 1 1 1-e 1-e 0+e],[0 0 1 1-e 0+e 0+e],c2);patch([0 0 1 1-e 0+e 0+e],[0 1 1 1-e 1-e 0+e],c3);plot([0 1 1 0 0],[0 0 1 1 0]);disp('Mux');
  dotprod1 : neural/Weight Functions/dotprod
  "lz{2,1}" : Outport
      mask Display: e = 0.06;c1 = [120 230 180]/255;c2 = ([120 230 180]+0)/(256+128);c3 = ([120 230 180]+128)/(256+128);patch([0 1 1 0],[0 0 1 1],c1);patch([0 1 1 1-e 1-e 0+e],[0 0 1 1-e 0+e 0+e],c2);patch([0 0 1 1-e 0+e 0+e],[0 1 1 1-e 1-e 0+e],c3);plot([0 1 1 0 0],[0 0 1 1 0]);
  wires:
  "IW{2,1}(1,:)'"/1 -> dotprod1/1
  "ad{2,1}"/1 -> dotprod1/2
  dotprod1/1 -> Mux/1
  Mux/1 -> "lz{2,1}"/1

== system plant_n/NARX Neural Network pretty gud/Layer 1/Delays 1 ==
  "p{1}" : Inport  PortDimensions=1  SampleTime=0.01
      mask Display: e = 0.06;c1 = [120 230 180]/255;c2 = ([120 230 180]+0)/(256+128);c3 = ([120 230 180]+128)/(256+128);patch([0 1 1 0],[0 0 1 1],c1);patch([0 1 1 1-e 1-e 0+e],[0 0 1 1-e 0+e 0+e],c2);patch([0 0 1 1-e 0+e 0+e],[0 1 1 1-e 1-e 0+e],c3);plot([0 1 1 0 0],[0 0 1 1 0]);
  Delay 1 : UnitDelay  InitialCondition=pi_input_1_delayed_1  SampleTime=0.01
      mask Display: e = 0.06;c1 = [120 150 230]/255;c2 = ([120 150 230]+0)/383;c3 = ([120 150 230]+128)/383;patch([0 1 1 0],[0 0 1 1],c1);patch([0 1 1 1-e 1-e 0+e],[0 0 1 1-e 0+e 0+e],c2);patch([0 0 1 1-e 0+e 0+e],[0 1 1 1-e 1-e 0+e],c3);plot([0 1 1 0 0],[0 0 1 1 0]);disp('D')
  Delay 2 : UnitDelay  InitialCondition=pi_input_1_delayed_2  SampleTime=0.01
      mask Display: e = 0.06;c1 = [120 150 230]/255;c2 = ([120 150 230]+0)/383;c3 = ([120 150 230]+128)/383;patch([0 1 1 0],[0 0 1 1],c1);patch([0 1 1 1-e 1-e 0+e],[0 0 1 1-e 0+e 0+e],c2);patch([0 0 1 1-e 0+e 0+e],[0 1 1 1-e 1-e 0+e],c3);plot([0 1 1 0 0],[0 0 1 1 0]);disp('D')
  Delay 3 : UnitDelay  InitialCondition=pi_input_1_delayed_3  SampleTime=0.01
      mask Display: e = 0.06;c1 = [120 150 230]/255;c2 = ([120 150 230]+0)/383;c3 = ([120 150 230]+128)/383;patch([0 1 1 0],[0 0 1 1],c1);patch([0 1 1 1-e 1-e 0+e],[0 0 1 1-e 0+e 0+e],c2);patch([0 0 1 1-e 0+e 0+e],[0 1 1 1-e 1-e 0+e],c3);plot([0 1 1 0 0],[0 0 1 1 0]);disp('D')
  Delay 4 : UnitDelay  InitialCondition=pi_input_1_delayed_4  SampleTime=0.01
      mask Display: e = 0.06;c1 = [120 150 230]/255;c2 = ([120 150 230]+0)/383;c3 = ([120 150 230]+128)/383;patch([0 1 1 0],[0 0 1 1],c1);patch([0 1 1 1-e 1-e 0+e],[0 0 1 1-e 0+e 0+e],c2);patch([0 0 1 1-e 0+e 0+e],[0 1 1 1-e 1-e 0+e],c3);plot([0 1 1 0 0],[0 0 1 1 0]);disp('D')
  Delay 5 : UnitDelay  InitialCondition=pi_input_1_delayed_5  SampleTime=0.01
      mask Display: e = 0.06;c1 = [120 150 230]/255;c2 = ([120 150 230]+0)/383;c3 = ([120 150 230]+128)/383;patch([0 1 1 0],[0 0 1 1],c1);patch([0 1 1 1-e 1-e 0+e],[0 0 1 1-e 0+e 0+e],c2);patch([0 0 1 1-e 0+e 0+e],[0 1 1 1-e 1-e 0+e],c3);plot([0 1 1 0 0],[0 0 1 1 0]);disp('D')
  Delay 6 : UnitDelay  InitialCondition=pi_input_1_delayed_6  SampleTime=0.01
      mask Display: e = 0.06;c1 = [120 150 230]/255;c2 = ([120 150 230]+0)/383;c3 = ([120 150 230]+128)/383;patch([0 1 1 0],[0 0 1 1],c1);patch([0 1 1 1-e 1-e 0+e],[0 0 1 1-e 0+e 0+e],c2);patch([0 0 1 1-e 0+e 0+e],[0 1 1 1-e 1-e 0+e],c3);plot([0 1 1 0 0],[0 0 1 1 0]);disp('D')
  Delay 7 : UnitDelay  InitialCondition=pi_input_1_delayed_7  SampleTime=0.01
      mask Display: e = 0.06;c1 = [120 150 230]/255;c2 = ([120 150 230]+0)/383;c3 = ([120 150 230]+128)/383;patch([0 1 1 0],[0 0 1 1],c1);patch([0 1 1 1-e 1-e 0+e],[0 0 1 1-e 0+e 0+e],c2);patch([0 0 1 1-e 0+e 0+e],[0 1 1 1-e 1-e 0+e],c3);plot([0 1 1 0 0],[0 0 1 1 0]);disp('D')
  mux : Mux  Inputs=7
      mask Display: e = 0.06;c1 = [120 150 230]/255;c2 = ([120 150 230]+0)/383;c3 = ([120 150 230]+128)/383;patch([0 1 1 0],[0 0 1 1],c1);patch([0 1 1 1-e 1-e 0+e],[0 0 1 1-e 0+e 0+e],c2);patch([0 0 1 1-e 0+e 0+e],[0 1 1 1-e 1-e 0+e],c3);plot([0 1 1 0 0],[0 0 1 1 0]);disp('Mux')
  "pd{1,1}" : Outport
      mask Display: e = 0.06;c1 = [120 230 180]/255;c2 = ([120 230 180]+0)/(256+128);c3 = ([120 230 180]+128)/(256+128);patch([0 1 1 0],[0 0 1 1],c1);patch([0 1 1 1-e 1-e 0+e],[0 0 1 1-e 0+e 0+e],c2);patch([0 0 1 1-e 0+e 0+e],[0 1 1 1-e 1-e 0+e],c3);plot([0 1 1 0 0],[0 0 1 1 0]);
  wires:
  "p{1}"/1 -> Delay 1/1
  Delay 1/1 -> Delay 2/1, mux/1
  Delay 2/1 -> Delay 3/1, mux/2
  Delay 3/1 -> Delay 4/1, mux/3
  Delay 4/1 -> Delay 5/1, mux/4
  Delay 5/1 -> Delay 6/1, mux/5
  Delay 6/1 -> Delay 7/1, mux/6
  Delay 7/1 -> mux/7
  mux/1 -> "pd{1,1}"/1
